simulink model "Workshop_0_44"  (R2019b)
settings: Solver=VariableStepAuto  StartTime=0.0  StopTime=10.0  RelTol=1e-3
libraries: dspsrcs4 x1
settings Model: Creator=linesLK  LastModifiedBy=linesLK

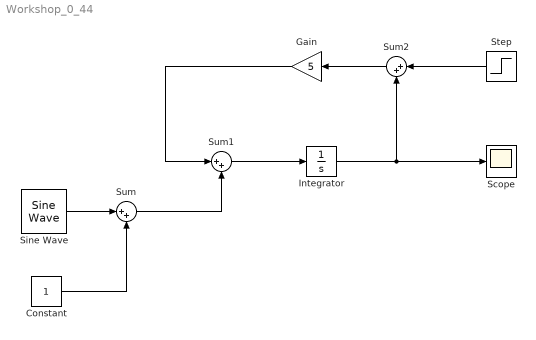
== system Workshop_0_44 ==
  Constant : Constant
  Gain : Gain  Gain=5
  Integrator : Integrator
  Scope : Scope
  Sine Wave : dspsrcs4/Sine Wave  Amplitude=1  Frequency=100  Phase=0  SampleMode=Continuous  OutComplex=Real  CompMethod=Trigonometric fcn  TableSize=Speed  SampleTime=1/1000  SamplesPerFrame=1  ResetState=Restart at time zero  OutputFrames=off  dataType=double  wordLen=16  udDataType=sfix(16)  fracBitsMode=Best precision  numFracBits=15  OutDataTypeStr=double  LastOutDataTypeStr=double
  Step : Step  SampleTime=0
  Sum : Sum  Inputs=|++
  Sum1 : Sum  Inputs=|++
  Sum2 : Sum  Inputs=|++
  wires:
  Sine Wave/1 -> Sum/1
  Constant/1 -> Sum/2
  Sum/1 -> Sum1/2
  Sum1/1 -> Integrator/1
  Sum2/1 -> Gain/1
  Step/1 -> Sum2/1
  Integrator/1 -> Sum2/2, Scope/1
  Gain/1 -> Sum1/1
